simulink model "regulator_po_stanjima"  (R2025a)
settings: Solver=VariableStepAuto  StartTime=0.0  StopTime=10  RelTol=1e-3
values from neighbouring files (symbols this model uses):
  A = [0, -1 ... (first row only)    [d2.m]
  B = [1; 0]    [d2.m]
  C = [1, 0]    [d2.m]
  D = 0    [d2.m]
  k = acker(A,B,[-5, -5])    [d2.m]
  kr = 1/(dcgain(Wsp0))    [d2.m]
  r = 10    [d2.m]
  x0 = [3 ... (first row only)    [d2.m]
settings Model: Creator=Korisnik  LastModifiedBy=Korisnik

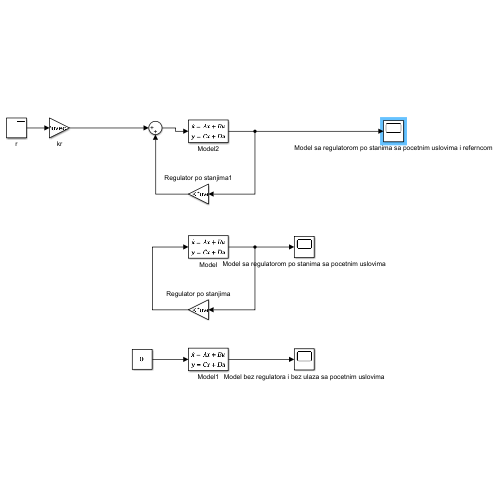
[thumbnail: Simulink's stored preview of the top-level diagram]
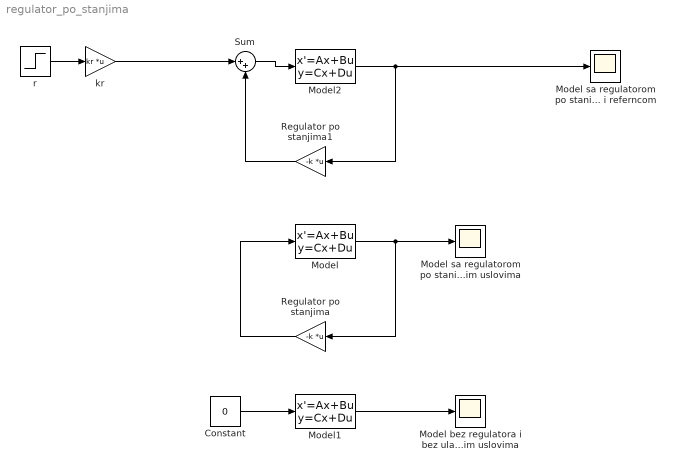
== system regulator_po_stanjima ==
  Constant : Constant  Value=0
  Model : StateSpace  A=A  B=B  C=[C; 0, 1]  D=[D;0]  InitialCondition=x0
  Model bez regulatora i bez ulaza sa pocetnim uslovima : Scope
      settings: ActiveDisplayYMinimum=-1  ActiveDisplayYMaximum=1
  Model sa regulatorom po stanima sa pocetnim uslovima : Scope
      settings: ActiveDisplayYMinimum=-1  ActiveDisplayYMaximum=1
  Model sa regulatorom po stanima sa pocetnim uslovima i referncom : Scope
      settings: ActiveDisplayYMinimum=-27.700648754597509  ActiveDisplayYMaximum=14.188960972733051  DataLoggingVariableName=ScopeData2
  Model1 : StateSpace  A=A  B=B  C=[C; 0, 1]  D=[D;0]  InitialCondition=x0
  Model2 : StateSpace  A=A  B=B  C=[C;0, 1]  D=[D;0]  InitialCondition=x0
  Regulator po stanjima : Gain  Gain=-k  Multiplication=Matrix(K*u) (u vector)
  Regulator po stanjima1 : Gain  Gain=-k  Multiplication=Matrix(K*u) (u vector)
  Sum : Sum  Inputs=|++
  kr : Gain  Gain=kr  Multiplication=Matrix(K*u) (u vector)
  r : Step  Time=0  Before=r  After=r  SampleTime=0
  wires:
  Model/1 -> Regulator po stanjima/1, Model sa regulatorom po stanima sa pocetnim uslovima/1
  Regulator po stanjima/1 -> Model/1
  Model1/1 -> Model bez regulatora i bez ulaza sa pocetnim uslovima/1
  Constant/1 -> Model1/1
  r/1 -> kr/1
  Model2/1 -> Regulator po stanjima1/1, Model sa regulatorom po stanima sa pocetnim uslovima i referncom/1
  Regulator po stanjima1/1 -> Sum/2
  Sum/1 -> Model2/1
  kr/1 -> Sum/1
